simulink model "Aufgabe_10_2_5_Drehteller"  (R2023a)
settings: Solver=ode3  StartTime=0.0  StopTime=40  FixedStep=0.01  RelTol=1e-3  EnableMultiTasking=on
undefined symbols (not defined in the file): A, I, igetr, K, MRK, PHI, Ra, U
libraries: simulink x5
settings Model: Creator=SimTP16  LastModifiedBy=ASUS
settings SolverCC: AlgebraicLoopSolver=TrustRegion
settings DataIOCC: LimitDataPoints=on  SaveFormat=Array  ReturnWorkspaceOutputs=off
settings OptimizationCC: LifeSpan=inf
settings DebuggingCC: UnderspecifiedInitializationDetection=Classic  MergeDetectMultiDrivingBlocksExec=none  SolverPrmCheckMsg=warning  UnconnectedInputMsg=warning  UnconnectedOutputMsg=warning  UnconnectedLineMsg=warning  StateNameClashWarn=warning  SFUnexpectedBacktrackingDiag=warning  SFNoUnconditionalDefaultTransitionDiag=warning  ArithmeticOperatorsInVariantConditions=warning
settings HardwareCC: ProdBitPerPointer=32  ProdBitPerSizeT=32  ProdBitPerPtrDiffT=32  ProdLargestAtomicFloat=None  ProdIntDivRoundTo=Undefined  ProdEndianess=Unspecified  ProdWordSize=32  ProdHWDeviceType=32-bit Generic
settings ModelReferenceCC: EnableRefExpFcnMdlSchedulingChecks=on  PropagateSignalLabelsOutOfModel=off
settings SFSimCC: SimUseLocalCustomCode=off  CustomCodeUndefinedFunction=UseInterfaceOnly
settings RTWCC: RTWUseLocalCustomCode=off
settings CodeAppCC: StateflowObjectComments=on
settings GRTTargetCC: TargetLangStandard=C89/C90 (ANSI)
settings ConfigComp: CovMetricSettings=dw  CovSaveCumulativeToWorkspaceVar=on  CovSaveSingleToWorkspaceVar=on  CovExternalEMLEnable=off

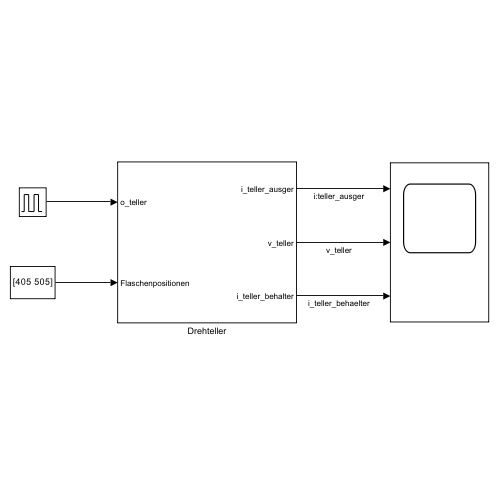
[thumbnail: Simulink's stored preview of the top-level diagram]
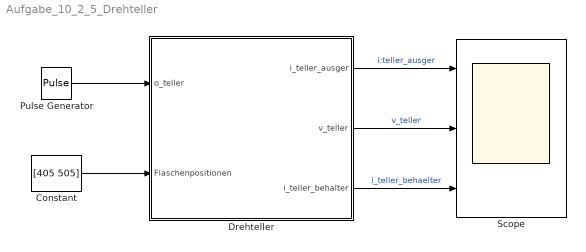
== system Aufgabe_10_2_5_Drehteller ==
  Constant : Constant  Value=[405 505]
  Drehteller : Subsystem
  Pulse Generator : DiscretePulseGenerator  PulseType=Time based  Period=3  PulseWidth=50
  Scope : Scope  NumInputPorts=3
  wires:
  Pulse Generator/1 -> Drehteller/1(o_teller)
  Constant/1 -> Drehteller/2(Flaschenpositionen)
  Drehteller/1(i_teller_ausger) -> Scope/1  "i:teller_ausger"
  Drehteller/2(v_teller) -> Scope/2  "v_teller"
  Drehteller/3(i_teller_behalter) -> Scope/3  "i_teller_behaelter"

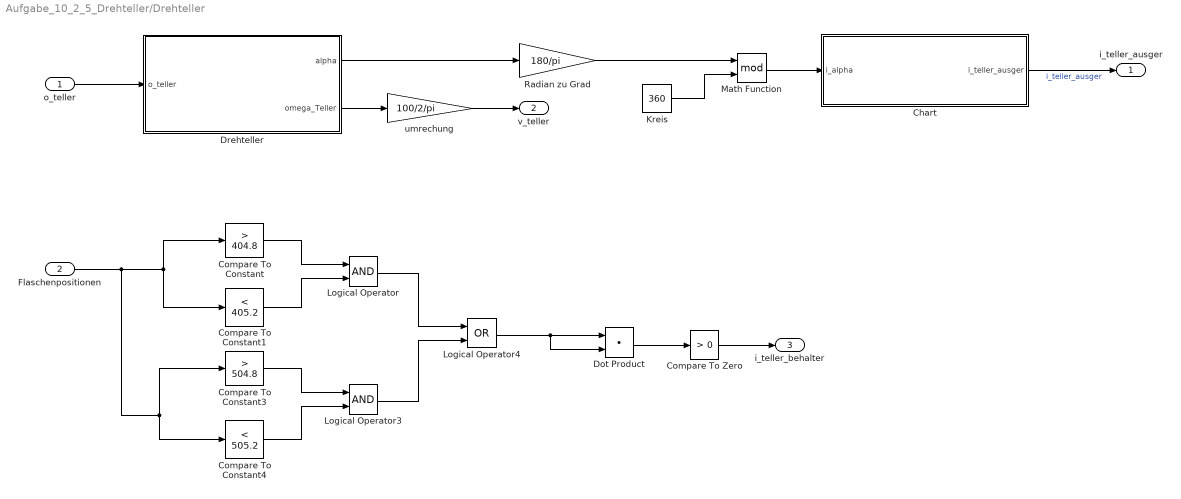
== system Aufgabe_10_2_5_Drehteller/Drehteller ==
  o_teller : Inport
  Flaschenpositionen : Inport  Port=2
  Chart : Stateflow chart  TreatAsAtomicUnit=on
  Compare To Constant : simulink/Logic and Bit Operations/Compare To Constant  relop=>  const=404.8  OutDataTypeStr=boolean
  Compare To Constant1 : simulink/Logic and Bit Operations/Compare To Constant  relop=<  const=405.2  OutDataTypeStr=boolean
  Compare To Constant3 : simulink/Logic and Bit Operations/Compare To Constant  relop=>  const=504.8  OutDataTypeStr=boolean
  Compare To Constant4 : simulink/Logic and Bit Operations/Compare To Constant  relop=<  const=505.2  OutDataTypeStr=boolean
  Compare To Zero : simulink/Logic and Bit Operations/Compare To Zero  relop=>  OutDataTypeStr=boolean
  Dot Product : DotProduct  OutDataTypeStr=Inherit: Inherit via internal rule
  Drehteller : Subsystem
  Kreis : Constant  Value=360
  Logical Operator : Logic  AllPortsSameDT=off  OutDataTypeStr=boolean
  Logical Operator3 : Logic  AllPortsSameDT=off  OutDataTypeStr=boolean
  Logical Operator4 : Logic  Operator=OR  AllPortsSameDT=off  OutDataTypeStr=boolean
  Math Function : Math  Operator=mod  SignedPower=on
  Radian zu Grad : Gain  Gain=180/pi
  umrechung : Gain  Gain=100/2/pi
  i_teller_ausger : Outport
  v_teller : Outport  Port=2
  i_teller_behalter : Outport  Port=3
  wires:
  Logical Operator4/1 -> Dot Product/2, Dot Product/1
  Dot Product/1 -> Compare To Zero/1
  Compare To Zero/1 -> i_teller_behalter/1
  Compare To Constant4/1 -> Logical Operator3/2
  Flaschenpositionen/1 -> Compare To Constant4/1, Compare To Constant3/1, Compare To Constant1/1, Compare To Constant/1
  Compare To Constant/1 -> Logical Operator/1
  Logical Operator/1 -> Logical Operator4/1
  Compare To Constant1/1 -> Logical Operator/2
  Logical Operator3/1 -> Logical Operator4/2
  Compare To Constant3/1 -> Logical Operator3/1
  o_teller/1 -> Drehteller/1(o_teller)
  Drehteller/2(omega_Teller) -> umrechung/1
  umrechung/1 -> v_teller/1
  Drehteller/1(alpha) -> Radian zu Grad/1
  Chart/1(i_teller_ausger) -> i_teller_ausger/1  "i_teller_ausger"
  Math Function/1 -> Chart/1(i_alpha)
  Radian zu Grad/1 -> Math Function/1
  Kreis/1 -> Math Function/2

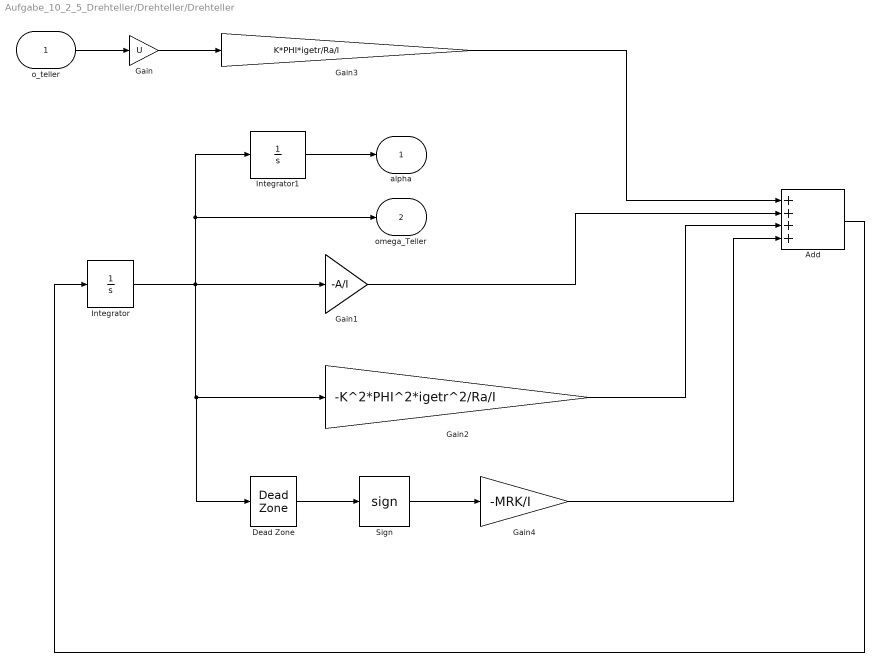
== system Aufgabe_10_2_5_Drehteller/Drehteller/Drehteller ==
  o_teller : Inport
  Add : Sum  Inputs=++++
  Dead Zone : DeadZone
  Gain : Gain  Gain=U
  Gain1 : Gain  Gain=-A/I
  Gain2 : Gain  Gain=-K^2*PHI^2*igetr^2/Ra/I
  Gain3 : Gain  Gain=K*PHI*igetr/Ra/I
  Gain4 : Gain  Gain=-MRK/I
  Integrator : Integrator
  Integrator1 : Integrator
  Sign : Signum
  alpha : Outport
  omega_Teller : Outport  Port=2
  wires:
  Integrator1/1 -> alpha/1
  Gain4/1 -> Add/4
  Sign/1 -> Gain4/1
  Dead Zone/1 -> Sign/1
  Gain2/1 -> Add/3
  Gain1/1 -> Add/2
  Gain3/1 -> Add/1
  Add/1 -> Integrator/1
  Integrator/1 -> omega_Teller/1, Integrator1/1, Dead Zone/1, Gain2/1, Gain1/1
  o_teller/1 -> Gain/1
  Gain/1 -> Gain3/1

== stateflow chart Aufgabe_10_2_5_Drehteller/Drehteller/Chart ==
  state Ausgerichtet
    en: i_teller_ausger = 1;
  state Nicht_ausgerichtet
    en: i_teller_ausger = 0;
  Nicht_ausgerichtet -> Ausgerichtet : [mod(i_alpha, 90) >88 || mod(i_alpha, 90) < 2]
  (default) -> Nicht_ausgerichtet
  Ausgerichtet -> Nicht_ausgerichtet : [mod(i_alpha, 90) >= 2 && mod(i_alpha, 90) <= 88]
  data: i_alpha input; i_teller_ausger output
